simulink model "PCM"  (R2015b)
settings: Solver=ode15s  StartTime=0.0  StopTime=tsim  FixedStep=0.0001  RelTol=1e-12  AbsTol=1e-12
undefined symbols (not defined in the file or in its folder): Per2
settings Model: Creator=AK69150  LastModifiedBy=lwoodward
settings DataIOCC: SaveFormat=Array  SignalLoggingSaveFormat=ModelDataLogs
settings DebuggingCC: UnderspecifiedInitializationDetection=Classic  MergeDetectMultiDrivingBlocksExec=none  SolverPrmCheckMsg=warning  MultiTaskDSMMsg=warning  MultiTaskCondExecSysMsg=none
settings HardwareCC: ProdBitPerPointer=32  ProdLargestAtomicFloat=None  ProdIntDivRoundTo=Undefined  ProdEndianess=Unspecified  ProdWordSize=32  ProdHWDeviceType=32-bit Generic
settings GRTTargetCC: GeneratePreprocessorConditionals=Disable all
settings ConfigComp: CovModelRefEnable=Off

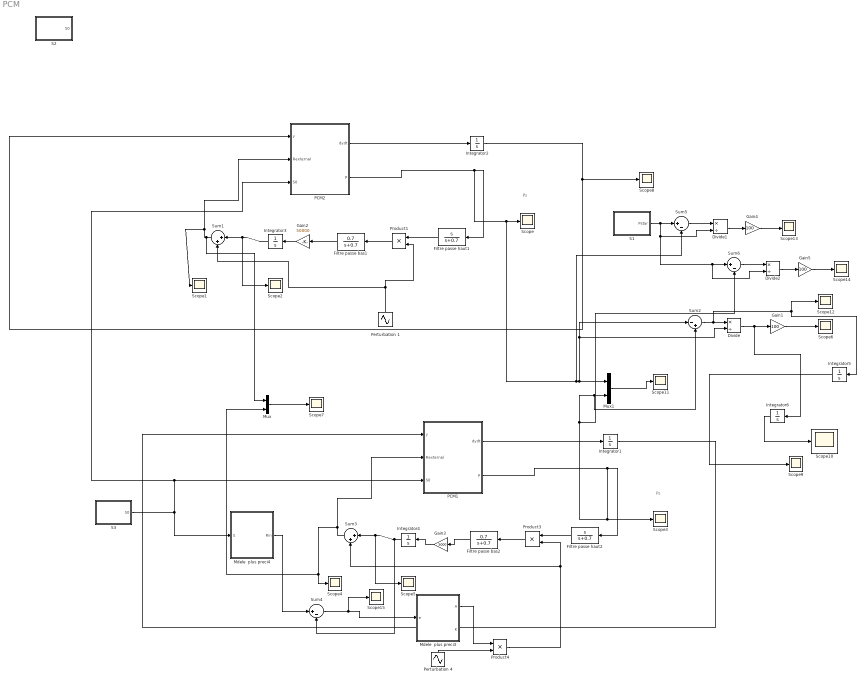
== system PCM ==
  note: Ps
  note: Ps
  Divide : Product  Inputs=*/
  Divide1 : Product  Inputs=*/
  Divide2 : Product  Inputs=*/
  Filtre passe bas1 : TransferFcn  Numerator=[0.7]  Denominator=[1 0.7]
  Filtre passe bas2 : TransferFcn  Numerator=[0.7]  Denominator=[1 0.7]
  Filtre passe haut1 : TransferFcn  Numerator=[1 0]  Denominator=[1 0.7]
  Filtre passe haut2 : TransferFcn  Numerator=[1 0]  Denominator=[1 0.7]
  Gain1 : Gain  Gain=100
  Gain2 : Gain  Gain=50000
  Gain3 : Gain  Gain=5000
  Gain4 : Gain  Gain=100
  Gain5 : Gain  Gain=100
  Integrator1 : Integrator  InitialCondition=[5.726117682433310 0.030299840936202]
  Integrator2 : Integrator  InitialCondition=[5.726117682433310 0.030299840936202]
  Integrator3 : Integrator  InitialCondition=157
  Integrator4 : Integrator  InitialCondition=157
  Integrator5 : Integrator
  Integrator6 : Integrator
  Mdele  plus preci3 : MATLAB Function  TreatAsAtomicUnit=on
  Mdele  plus preci4 : MATLAB Function  TreatAsAtomicUnit=on
  Mux : Mux  Inputs=2
  Mux1 : Mux  Inputs=2
  PCM1 : MATLAB Function  TreatAsAtomicUnit=on
  PCM2 : MATLAB Function  TreatAsAtomicUnit=on
  Perturbation 1 : Sin  Amplitude=2  Frequency=3.8  SampleTime=0
  Perturbation 4 : Sin  Frequency=3.8  SampleTime=0
  Product1 : Product  RndMeth=Zero
  Product3 : Product  RndMeth=Zero
  Product4 : Product  RndMeth=Zero
  S1 : Subsystem
  S2 : Subsystem
  S3 : Subsystem
  Scope{,1..15} (16 alike) : Scope
  Sum1 : Sum  Inputs=|++
  Sum2 : Sum  Inputs=|-+
  Sum3 : Sum  Inputs=|++
  Sum4 : Sum  Inputs=|+-
  Sum5 : Sum  Inputs=|+-
  Sum6 : Sum  Inputs=|+-
  wires:
  Integrator2/1 -> PCM2/1(y), Scope8/1
  PCM2/1(dydt) -> Integrator2/1
  PCM2/2(P) -> Sum5/2, Divide/2, Sum2/1, Mux1/1, Scope/1, Filtre passe haut1/1
  Product1/1 -> Filtre passe bas1/1
  Integrator3/1 -> Scope2/1, Sum1/1
  Gain2/1 -> Integrator3/1
  Filtre passe bas1/1 -> Gain2/1
  Filtre passe haut1/1 -> Product1/1
  Sum1/1 -> Mux/1, PCM2/2(Rexternal), Scope1/1
  Integrator1/1 -> PCM1/1(y)
  PCM1/1(dydt) -> Integrator1/1
  Product3/1 -> Filtre passe bas2/1
  Integrator4/1 -> Sum4/2, Scope5/1, Sum3/1
  Gain3/1 -> Integrator4/1
  Filtre passe bas2/1 -> Gain3/1
  Filtre passe haut2/1 -> Product3/1
  Sum3/1 -> PCM1/2(Rexternal), Mux/2, Scope4/1
  Mdele  plus preci4/1(Rin) -> Sum4/1
  Sum4/1 -> Scope15/1, Mdele  plus preci3/1(e)
  Perturbation 4/1 -> Product4/2
  Mdele  plus preci3/1(A) -> Product4/1
  Product4/1 -> Sum3/2, Product3/2
  Perturbation 1/1 -> Sum1/2, Product1/2
  Mux/1 -> Scope7/1
  Mux1/1 -> Scope11/1
  S3/1(S0) -> PCM2/3(S0), PCM1/3(S0), Mdele  plus preci4/1(S)
  Sum2/1 -> Scope12/1, Integrator5/1, Divide/1
  Divide/1 -> Integrator6/1, Gain1/1
  Gain1/1 -> Scope6/1
  Sum5/1 -> Divide1/1
  Divide1/1 -> Gain4/1
  Gain4/1 -> Scope13/1
  PCM1/2(P) -> Scope3/1, Sum6/2, Sum2/2, Mux1/2, Filtre passe haut2/1
  S1/1(Pstar) -> Divide2/2, Sum6/1, Divide1/2, Sum5/1
  Sum6/1 -> Divide2/1
  Divide2/1 -> Gain5/1
  Gain5/1 -> Scope14/1
  Integrator5/1 -> Scope9/1
  Integrator6/1 -> Scope10/1

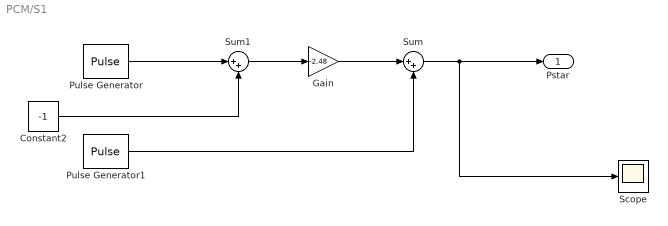
== system PCM/S1 ==
  Constant2 : Constant  Value=-1
  Gain : Gain  Gain=-2.48
  Pulse Generator : DiscretePulseGenerator  PulseType=Time based  Period=Per2  PulseWidth=50
  Pulse Generator1 : DiscretePulseGenerator  PulseType=Time based  Amplitude=1.47  Period=Per2  PulseWidth=50
  Scope : Scope
  Sum : Sum  Inputs=|++
  Sum1 : Sum  Inputs=|++
  Pstar : Outport
  wires:
  Pulse Generator/1 -> Sum1/1
  Pulse Generator1/1 -> Sum/2
  Constant2/1 -> Sum1/2
  Sum1/1 -> Gain/1
  Gain/1 -> Sum/1
  Sum/1 -> Pstar/1, Scope/1

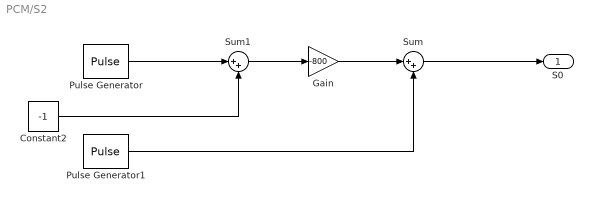
== system PCM/S2 ==
  Constant2 : Constant  Value=-1
  Gain : Gain  Gain=-800
  Pulse Generator : DiscretePulseGenerator  PulseType=Time based  Period=7  PulseWidth=50
  Pulse Generator1 : DiscretePulseGenerator  PulseType=Time based  Amplitude=300  Period=7  PulseWidth=50
  Sum : Sum  Inputs=|++
  Sum1 : Sum  Inputs=|++
  S0 : Outport
  wires:
  Pulse Generator/1 -> Sum1/1
  Pulse Generator1/1 -> Sum/2
  Constant2/1 -> Sum1/2
  Sum1/1 -> Gain/1
  Gain/1 -> Sum/1
  Sum/1 -> S0/1

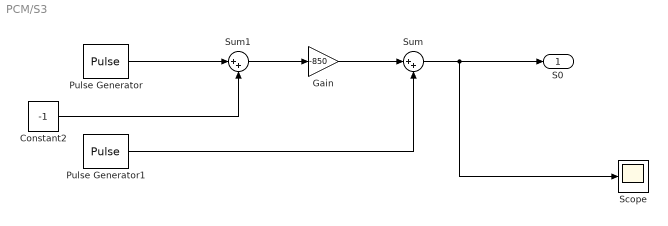
== system PCM/S3 ==
  Constant2 : Constant  Value=-1
  Gain : Gain  Gain=-850
  Pulse Generator : DiscretePulseGenerator  PulseType=Time based  Period=Per2  PulseWidth=50
  Pulse Generator1 : DiscretePulseGenerator  PulseType=Time based  Amplitude=350  Period=Per2  PulseWidth=50
  Scope : Scope
  Sum : Sum  Inputs=|++
  Sum1 : Sum  Inputs=|++
  S0 : Outport
  wires:
  Pulse Generator/1 -> Sum1/1
  Pulse Generator1/1 -> Sum/2
  Constant2/1 -> Sum1/2
  Sum1/1 -> Gain/1
  Gain/1 -> Sum/1
  Sum/1 -> S0/1, Scope/1

== matlab function PCM/Mdele  plus preci3 ==
  data: e input; A output; K output
function [A,K] = fcn(e)


if abs(e)>10
    A=20;
    K=5000;

else
    A=2;
  K=50000;
end

== matlab function PCM/Mdele  plus preci4 ==
  data: S input; Rin output
function Rin = fcn(S)

W1= [-3.3685    2.5640    0.3670   -4.7976   -0.8754   -1.3498    0.5468    0.4064    0.6063    2.9323; -16.9080   -2.1163   -0.3142    6.2725    0.7329    1.0987   -0.4653   -0.3477   -0.5147   -2.6463];
W2=[ 9.8215
    4.4782
   -0.0111
    0.1037
   -0.4259
   -0.2185
   -0.2740
    0.1494
    0.1140
    0.1634
   -0.4299];
a=.5;%pente de la sigmoide

in=0.001*S;

Y0=[.5 in]';
U1=W1'*Y0;
Y1=(1-exp(-a*U1))./(1+exp(-a*U1));
Y2=[0.5;Y1];
U2=W2'*Y2;
Y3=(1-exp(-a*U2))./(1+exp(-a*U2));
Rin=Y3/0.001;

== matlab function PCM/PCM2 ==
  data: y input; dydt output; Rexternal input; S0 input; P output

function [dydt,P]=fcnn(y,Rexternal,S0)

yield = 22.753;      %constant [ ] OK
F=96485;                 %Faraday constant [A.s/mol] OK
Emin= 0.01;             % Minimum cell voltage [V] OK
qmax1=2.1210*4;         %max S consumption rate [1/day] OK
qmax2=2.05*4;                %max S consumption rate [1/day] OK
Ks1=20;                   %constant Substrate/Electrogens  [mg/L] OK
Ks2=80;                 %constant Substrate/Methanogens  [mg/L] OK
m=2;                        %constant, e- mols tranferd [mol] OK
Mtotal=0.05;                 %mediator concentration (Mred+Mox) per microorganism (Mox+Mred=Const) [mg-M/mg-Xeg] OK
Km=0.2*Mtotal;          % Monod term for Mox limitation (per microorganism) OK
eps=0.0001*Mtotal;       % limitation constant to avoid current generation in Faraday's law (when Mred->0)

Kx=0.01*4;              % detachment+death constant OK
umax1=1.9753;                 %Electrogens max grow rate [1/day] OK
umax2=0.1;                 %Methanogens max grow rate [1/day] OK
Y2=0.3;                        %Methane balance relationship with methanogens concentration OK
Xmax=2050/4;                 %Maximum concentration of Biomass in the Biofilm - Space limitation
% Xmax2=2150/4;                 %Maximum concentration of Biomass in the Biofilm - Space limitation 525!!!
% Xmax2=525;                 %Maximum concentration of Biomass in the Biofilm - Space limitation 525!!!
Kd1=0.02*umax1;                  %Decaing constant for Xeg OK
Kd2=0.02*umax2;                   %Decaing constant for Xmth OK
R=8.314472;              %gas ideal constant [J/K.mol] OK
T=298.15;                %Temperrature [K] OK
gamma=663400;            %NADP molar weight [mg/mol] OK
Kr=0.006*4;                 % Internal resistance constant 0,006!!!
% Kr=0.006;
Rmin=25;                  % Minimum value of Internal resistance OK
Rmax=2000+Rmin;                % Maximum value of Internal resistance 2000!!!
Emax=0.25 + 0.4144+ Emin; %OK
i0ref=0.4*4; 
time = 0.2;
V = 0.2;
Flow = 0.1527;

Xtot = 500;

Xeg = 250;


S = y(1);
% Xeg = x(2,:);
% Xmth = x(3,:);
Mox = y(2);
Xmth = Xtot-Xeg;
%Definitions
Mred = Mtotal-Mox;
Rint = Rmin+(Rmax-Rmin)*exp(-Kr*Xeg);
Ethermo = Emin + (Emax-Emin)*exp(-1/(Kr*Xeg));
alpha = (1+tanh(Kx*((Xeg+Xmth)-Xmax)))/2;
% alpha2 = (1+tanh(Kx*((Xeg+Xmth)-Xmax2)))/2;


%Reaction rates
qeg = qmax1*(S/(Ks1+S))*(Mox/(Km+Mox));                                    %Substrate X Electrogens
qmth = qmax2*(S/(Ks2+S));                                                        %Substrate X Methanogens
Ueg = umax1*(S/(Ks1+S))*(Mox/(Km+Mox));   %Electrogens
% Umth = umax2*(S/(Ks2+S));                       %Methanogens
  
%Icell1 = (Ethermo - (R *T /m /F)*log(Mtotal/Mred))/(Rexternal + Rint)*Mred/(eps+Mred);



Mredvec = Mtotal-y(2);

Rintvec = Rmin+(Rmax-Rmin)*exp(-Kr*Xeg);

Ethermovec = Emin + (Emax-Emin)*exp(-1/(Kr*Xeg));

Icell1vec = (Ethermovec - (R *T /m /F)*abs(log(complex(Mtotal/Mredvec))))/(Rexternal + Rintvec)*Mredvec/(eps+Mredvec);

RintVerif = ((Ethermovec - (R *T /m /F)*abs(log(complex(Mtotal/Mredvec))))*Mredvec/(eps+Mredvec))/Icell1vec-Rexternal;

Ps= Rexternal*Icell1vec*Icell1vec;


P= ((Ethermovec - (R *T /m /F)*abs(log(complex(Mtotal/Mredvec))))*Mredvec/(eps+Mredvec)-Rintvec*Icell1vec)*Icell1vec;

% Mass Balances 
dSdt = -qeg*Xeg - qmth*Xmth + Flow/V*(S0-S);  
% dXegdt = (Ueg - Kd1)*Xeg - alpha*Flow/V*Xeg;
% dXmthdt = (Umth - Kd2)*Xmth - alpha2*Flow/V*Xmth; 
dMoxdt = -yield*qeg + gamma*Icell1vec/m/F*86400/Xeg/V;






dydt=[dSdt dMoxdt];

== matlab function PCM/PCM1 ==
  data: y input; dydt output; Rexternal input; S0 input; P output

function [dydt,P]=fcnn(y,Rexternal,S0)

yield = 22.753;      %constant [ ] OK
F=96485;                 %Faraday constant [A.s/mol] OK
Emin= 0.01;             % Minimum cell voltage [V] OK
qmax1=2.1210*4;         %max S consumption rate [1/day] OK
qmax2=2.05*4;                %max S consumption rate [1/day] OK
Ks1=20;                   %constant Substrate/Electrogens  [mg/L] OK
Ks2=80;                 %constant Substrate/Methanogens  [mg/L] OK
m=2;                        %constant, e- mols tranferd [mol] OK
Mtotal=0.05;                 %mediator concentration (Mred+Mox) per microorganism (Mox+Mred=Const) [mg-M/mg-Xeg] OK
Km=0.2*Mtotal;          % Monod term for Mox limitation (per microorganism) OK
eps=0.0001*Mtotal;       % limitation constant to avoid current generation in Faraday's law (when Mred->0)

Kx=0.01*4;              % detachment+death constant OK
umax1=1.9753;                 %Electrogens max grow rate [1/day] OK
umax2=0.1;                 %Methanogens max grow rate [1/day] OK
Y2=0.3;                        %Methane balance relationship with methanogens concentration OK
Xmax=2050/4;                 %Maximum concentration of Biomass in the Biofilm - Space limitation
% Xmax2=2150/4;                 %Maximum concentration of Biomass in the Biofilm - Space limitation 525!!!
% Xmax2=525;                 %Maximum concentration of Biomass in the Biofilm - Space limitation 525!!!
Kd1=0.02*umax1;                  %Decaing constant for Xeg OK
Kd2=0.02*umax2;                   %Decaing constant for Xmth OK
R=8.314472;              %gas ideal constant [J/K.mol] OK
T=298.15;                %Temperrature [K] OK
gamma=663400;            %NADP molar weight [mg/mol] OK
Kr=0.006*4;                 % Internal resistance constant 0,006!!!
% Kr=0.006;
Rmin=25;                  % Minimum value of Internal resistance OK
Rmax=2000+Rmin;                % Maximum value of Internal resistance 2000!!!
Emax=0.25 + 0.4144+ Emin; %OK
i0ref=0.4*4; 
time = 0.2;
V = 0.2;
Flow = 0.1527;

Xtot = 500;

Xeg = 250;


S = y(1);
% Xeg = x(2,:);
% Xmth = x(3,:);
Mox = y(2);
Xmth = Xtot-Xeg;
%Definitions
Mred = Mtotal-Mox;
Rint = Rmin+(Rmax-Rmin)*exp(-Kr*Xeg);
Ethermo = Emin + (Emax-Emin)*exp(-1/(Kr*Xeg));
alpha = (1+tanh(Kx*((Xeg+Xmth)-Xmax)))/2;
% alpha2 = (1+tanh(Kx*((Xeg+Xmth)-Xmax2)))/2;


%Reaction rates
qeg = qmax1*(S/(Ks1+S))*(Mox/(Km+Mox));                                    %Substrate X Electrogens
qmth = qmax2*(S/(Ks2+S));                                                        %Substrate X Methanogens
Ueg = umax1*(S/(Ks1+S))*(Mox/(Km+Mox));   %Electrogens
% Umth = umax2*(S/(Ks2+S));                       %Methanogens
  
%Icell1 = (Ethermo - (R *T /m /F)*log(Mtotal/Mred))/(Rexternal + Rint)*Mred/(eps+Mred);



Mredvec = Mtotal-y(2);

Rintvec = Rmin+(Rmax-Rmin)*exp(-Kr*Xeg);

Ethermovec = Emin + (Emax-Emin)*exp(-1/(Kr*Xeg));

Icell1vec = (Ethermovec - (R *T /m /F)*abs(log(complex(Mtotal/Mredvec))))/(Rexternal + Rintvec)*Mredvec/(eps+Mredvec);

RintVerif = ((Ethermovec - (R *T /m /F)*abs(log(complex(Mtotal/Mredvec))))*Mredvec/(eps+Mredvec))/Icell1vec-Rexternal;

Ps= Rexternal*Icell1vec*Icell1vec;


P= ((Ethermovec - (R *T /m /F)*abs(log(complex(Mtotal/Mredvec))))*Mredvec/(eps+Mredvec)-Rintvec*Icell1vec)*Icell1vec;

% Mass Balances 
dSdt = -qeg*Xeg - qmth*Xmth + Flow/V*(S0-S);  
% dXegdt = (Ueg - Kd1)*Xeg - alpha*Flow/V*Xeg;
% dXmthdt = (Umth - Kd2)*Xmth - alpha2*Flow/V*Xmth; 
dMoxdt = -yield*qeg + gamma*Icell1vec/m/F*86400/Xeg/V;


dydt=[dSdt dMoxdt];
